simulink library "GOcontroll_Generic"  (R2023b)
settings: Solver=ode45  StartTime=0.0  StopTime=10.0  RelTol=1e-3  EnableMultiTasking=on
undefined symbols (not defined in the file or in its folder): C_CatOutPos, C_Cb1Pt10, Cb1Pt10_RAW_ERR_HIGH, Cb1Pt10_RAW_ERR_LOW, Cb1Pt10_SIG_ERR_HIGH, Cb1Pt10_SIG_ERR_LOW, Cb1Pt10_SIG_WAR_HIGH, Cb1Pt10_SIG_WAR_LOW, M_CatOutPos, Pres_0_20_bar_500_4500_mv_inv, SensorSignalSimulation, signal_x_RAW_ERR_HIGH, signal_x_RAW_ERR_LOW, signal_x_SIG_ERR_HIGH, signal_x_SIG_ERR_LOW, signal_x_SIG_WAR_HIGH, signal_x_SIG_WAR_LOW, signal_x_SPN, Valve1_ACTIVE_DUTY_CYCLE, Valve1_MAX_CURRENT, Valve1_MIN_CURRENT, Valve1_SPN
libraries: simulink x23, GOcontroll_Moduline_Target x20
(part 2 of 2)

== stateflow chart GOcontroll_Generic/Plausability Checks/H2 PPM Diagnose 2 Levels/Chart4 ==
  state Entry
    en:SetDiagnosticCode = 0;
  state System_Running
  state Error_Triggered
  state Error_Triggered_Confirmed
    en:SetDiagnosticCode = 1;
  state Error_Code_Stored
    en:SetDiagnosticCode = 0;
  (default) -> Entry
  Entry -> System_Running : [after(StartupDelayMs,msec)]
  Error_Triggered -> System_Running [order 2] : [Trigger == 0]
  Error_Code_Stored -> System_Running
  System_Running -> Error_Triggered : [Trigger == 1]
  Error_Triggered -> Error_Triggered_Confirmed [order 1] : [after(TriggerDurationMs,msec)]
  Error_Triggered_Confirmed -> Error_Code_Stored : [after(1,sec)]
  data: Trigger input; StartupDelayMs input single; TriggerDurationMs input single; SetDiagnosticCode output uint8

== stateflow chart GOcontroll_Generic/Plausability Checks/Actuator No//Low Current Detection/Chart ==
  state Entry
    en:SetDiagnosticCode = 0;
  state Valve_Actuating
  state Current_Flowing
  state No_Valve_Current
    en:SetDiagnosticCode = 1;
  state Valve_Actuated
  (default) -> Entry
  Valve_Actuated -> Entry [order 2] : [ValveState==0]
  Current_Flowing -> Entry [order 3] : [ValveState==0]
  Valve_Actuating -> Entry [order 1] : [ValveState==0]
  Entry -> Valve_Actuating : [ValveState==1]
  Valve_Actuating -> Current_Flowing [order 2] : [after(100,msec)]
  Current_Flowing -> No_Valve_Current [order 2] : [after(100,msec)]
  Current_Flowing -> Valve_Actuated [order 1] : [ValveCurrent>=MinimalActuatedValveCurrent]
  Valve_Actuated -> No_Valve_Current [order 1] : [ValveCurrent<MinimalActuatedValveCurrent && ValveState==1]
  data: ValveState input; ValveCurrent input; SetDiagnosticCode output; MinimalActuatedValveCurrent parameter

== stateflow chart GOcontroll_Generic/Diagnostic checks/Actuator diagnostic/Chart1 ==
  state Entry
    en:SetDiagnosticCode = 0;
    en:FlagPersist = uint8(0);
    en:FlagVolatile = uint8(0);
  state Reset_Flag
    state System_Running
      en:FlagVolatile = 0;
    state Error_Triggered
    state Error_Triggered_Confirmed
      en:SetDiagnosticCode = 1;
      en:FlagPersist = 1;
      en:FlagVolatile = 1;
    state Error_Code_Stored
      en:SetDiagnosticCode = 0;
    System_Running -> Error_Triggered : [Trigger == 1]
    Error_Triggered -> System_Running [order 2] : [Trigger == 0]
    Error_Code_Stored -> System_Running : [Trigger == 0]
    Error_Triggered -> Error_Triggered_Confirmed [order 1] : [after(duration,msec)]
    Error_Triggered_Confirmed -> Error_Code_Stored : [after(1,sec)]
  (default) -> Entry
  Entry -> System_Running : [after(delay,msec)]
  Reset_Flag -> Entry : [Reset == 1]
  data: Reset input; FlagPersist output; FlagVolatile output; Trigger input; SetDiagnosticCode output uint8; delay parameter single; duration parameter single

== stateflow chart GOcontroll_Generic/Plausability Checks/Actuator short circuit//over current detection/Chart ==
  state DefaultState
    en:SetFaultCode = 0;
  state AlertState
  state ErrorState
    en:SetFaultCode = 1;
  (default) -> DefaultState
  AlertState -> DefaultState [order 1] : [Trigger==0]
  DefaultState -> AlertState : [Trigger==1]
  AlertState -> ErrorState [order 2] : [after(2,sec)]
  data: Trigger input; SetFaultCode output

== stateflow chart GOcontroll_Generic/Plausability Checks/Actuator short circuit//over current detection/Chart1 ==
  state DefaultState
    en:SetFaultCode = 0;
  state AlertState
  state ErrorState
    en:SetFaultCode = 1;
  (default) -> DefaultState
  AlertState -> DefaultState [order 1] : [Trigger==0]
  DefaultState -> AlertState : [Trigger==1]
  AlertState -> ErrorState [order 2] : [after(2,sec)]
  data: Trigger input; SetFaultCode output

== stateflow chart GOcontroll_Generic/Diagnostic checks/Actuator diagnostic/Chart4 ==
  state Entry
    en:SetDiagnosticCode = 0;
    en:FlagPersist = uint8(0);
    en:FlagVolatile = uint8(0);
  state Reset_Flag
    state System_Running
      en:FlagVolatile = 0;
    state Error_Triggered
    state Error_Triggered_Confirmed
      en:SetDiagnosticCode = 1;
      en:FlagPersist = 1;
      en:FlagVolatile = 1;
    state Error_Code_Stored
      en:SetDiagnosticCode = 0;
    System_Running -> Error_Triggered : [Trigger == 1]
    Error_Triggered -> System_Running [order 2] : [Trigger == 0]
    Error_Code_Stored -> System_Running : [Trigger == 0]
    Error_Triggered -> Error_Triggered_Confirmed [order 1] : [after(duration,msec)]
    Error_Triggered_Confirmed -> Error_Code_Stored : [after(1,sec)]
  (default) -> Entry
  Entry -> System_Running : [after(delay,msec)]
  Reset_Flag -> Entry : [Reset == 1]
  data: Reset input; FlagPersist output; FlagVolatile output; Trigger input; SetDiagnosticCode output uint8; delay parameter single; duration parameter single

== stateflow chart GOcontroll_Generic/Diagnostic checks/Generic diagnostic/Chart4 ==
  state Entry
    en:SetDiagnosticCode = 0;
    en:FlagPersist = uint8(0);
    en:FlagVolatile = uint8(0);
  state Reset_Flag
    state System_Running
      en:FlagVolatile = 0;
    state Error_Triggered
    state Error_Triggered_Confirmed
      en:SetDiagnosticCode = 1;
      en:FlagPersist = 1;
      en:FlagVolatile = 1;
    state Error_Code_Stored
      en:SetDiagnosticCode = 0;
    System_Running -> Error_Triggered : [Trigger == 1]
    Error_Triggered -> System_Running [order 2] : [Trigger == 0]
    Error_Code_Stored -> System_Running : [Trigger == 0]
    Error_Triggered -> Error_Triggered_Confirmed [order 1] : [after(duration,msec)]
    Error_Triggered_Confirmed -> Error_Code_Stored : [after(1,sec)]
  (default) -> Entry
  Entry -> System_Running : [after(delay,msec)]
  Reset_Flag -> Entry : [Reset == 1]
  data: Reset input; FlagPersist output; FlagVolatile output; Trigger input; SetDiagnosticCode output uint8; delay parameter single; duration parameter single

== stateflow chart GOcontroll_Generic/Plausability Checks/Tank Pressure & Temp Diagnostic Block/Chart10 ==
  state Entry
    en:SetDiagnosticCode = 0;
  state System_Running
  state Error_Triggered
  state Error_Triggered_Confirmed
    en:SetDiagnosticCode = 1;
  state Error_Code_Stored
    en:SetDiagnosticCode = 0;
  (default) -> Entry
  Entry -> System_Running : [after(StartupDelayMs,msec)]
  Error_Triggered -> System_Running [order 2] : [Trigger == 0]
  Error_Code_Stored -> System_Running
  System_Running -> Error_Triggered : [Trigger == 1]
  Error_Triggered -> Error_Triggered_Confirmed [order 1] : [after(TriggerDurationMs,msec)]
  Error_Triggered_Confirmed -> Error_Code_Stored : [after(1,sec)]
  data: Trigger input; StartupDelayMs input single; TriggerDurationMs input single; SetDiagnosticCode output uint8

== stateflow chart GOcontroll_Generic/Diagnostic checks/Signal diagnostic/Chart1 ==
  state Entry
    en:SetDiagnosticCode = 0;
    en:FlagPersist = 0;
    en:FlagVolatile = 0;
  state Reset_Flag
    state System_Running
      en:FlagVolatile = 0;
    state Error_Triggered
    state Error_Triggered_Confirmed
      en:SetDiagnosticCode = 1;
      en:FlagPersist = 1;
      en:FlagVolatile = 1;
    state Error_Code_Stored
      en:SetDiagnosticCode = 0;
    System_Running -> Error_Triggered : [Trigger == 1]
    Error_Triggered -> System_Running [order 2] : [Trigger == 0]
    Error_Code_Stored -> System_Running : [Trigger == 0]
    Error_Triggered -> Error_Triggered_Confirmed [order 1] : [after(duration,msec)]
    Error_Triggered_Confirmed -> Error_Code_Stored : [after(1,sec)]
  (default) -> Entry
  Entry -> System_Running : [after(delay,msec)]
  Reset_Flag -> Entry : [Reset == 1]
  data: Reset input; FlagPersist output; FlagVolatile output; Trigger input; SetDiagnosticCode output uint8; delay parameter single; duration parameter single

== stateflow chart GOcontroll_Generic/Plausability Checks/Chart4 ==
  state Entry
    en:SetDiagnosticCode = 0;
  state System_Running
  state Error_Triggered
  state Error_Triggered_Confirmed
    en:SetDiagnosticCode = 1;
  state Error_Code_Stored
    en:SetDiagnosticCode = 0;
  (default) -> Entry
  Entry -> System_Running : [after(StartupDelayMs,msec)]
  Error_Triggered -> System_Running [order 2] : [Trigger == 0]
  Error_Code_Stored -> System_Running
  System_Running -> Error_Triggered : [Trigger == 1]
  Error_Triggered -> Error_Triggered_Confirmed [order 1] : [after(TriggerDurationMs,msec)]
  Error_Triggered_Confirmed -> Error_Code_Stored : [after(1,sec)]
  data: Trigger input; StartupDelayMs input single; TriggerDurationMs input single; SetDiagnosticCode output uint8

== stateflow chart GOcontroll_Generic/Diagnostic checks/Signal diagnostic/Chart2 ==
  state Entry
    en:SetDiagnosticCode = 0;
    en:FlagPersist = 0;
    en:FlagVolatile = 0;
  state Reset_Flag
    state System_Running
      en:FlagVolatile = 0;
    state Error_Triggered
    state Error_Triggered_Confirmed
      en:SetDiagnosticCode = 1;
      en:FlagPersist = 1;
      en:FlagVolatile = 1;
    state Error_Code_Stored
      en:SetDiagnosticCode = 0;
    System_Running -> Error_Triggered : [Trigger == 1]
    Error_Triggered -> System_Running [order 2] : [Trigger == 0]
    Error_Code_Stored -> System_Running : [Trigger == 0]
    Error_Triggered -> Error_Triggered_Confirmed [order 1] : [after(duration,msec)]
    Error_Triggered_Confirmed -> Error_Code_Stored : [after(1,sec)]
  (default) -> Entry
  Entry -> System_Running : [after(delay,msec)]
  Reset_Flag -> Entry : [Reset == 1]
  data: Reset input; FlagPersist output; FlagVolatile output; Trigger input; SetDiagnosticCode output uint8; delay parameter single; duration parameter single

== stateflow chart GOcontroll_Generic/Diagnostic checks/Signal diagnostic/Chart3 ==
  state Entry
    en:SetDiagnosticCode = 0;
    en:FlagPersist = 0;
    en:FlagVolatile = 0;
  state Reset_Flag
    state System_Running
      en:FlagVolatile = 0;
    state Error_Triggered
    state Error_Triggered_Confirmed
      en:SetDiagnosticCode = 1;
      en:FlagPersist = 1;
      en:FlagVolatile = 1;
    state Error_Code_Stored
      en:SetDiagnosticCode = 0;
    System_Running -> Error_Triggered : [Trigger == 1]
    Error_Triggered -> System_Running [order 2] : [Trigger == 0]
    Error_Code_Stored -> System_Running : [Trigger == 0]
    Error_Triggered -> Error_Triggered_Confirmed [order 1] : [after(duration,msec)]
    Error_Triggered_Confirmed -> Error_Code_Stored : [after(1,sec)]
  (default) -> Entry
  Entry -> System_Running : [after(delay,msec)]
  Reset_Flag -> Entry : [Reset == 1]
  data: Reset input; FlagPersist output; FlagVolatile output; Trigger input; SetDiagnosticCode output uint8; delay parameter single; duration parameter single

== stateflow chart GOcontroll_Generic/Diagnostic checks/Signal diagnostic/Chart4 ==
  state Entry
    en:SetDiagnosticCode = 0;
    en:FlagPersist = 0;
    en:FlagVolatile = 0;
  state Reset_Flag
    state System_Running
      en:FlagVolatile = 0;
    state Error_Triggered
    state Error_Triggered_Confirmed
      en:SetDiagnosticCode = 1;
      en:FlagPersist = 1;
      en:FlagVolatile = 1;
    state Error_Code_Stored
      en:SetDiagnosticCode = 0;
    System_Running -> Error_Triggered : [Trigger == 1]
    Error_Triggered -> System_Running [order 2] : [Trigger == 0]
    Error_Code_Stored -> System_Running : [Trigger == 0]
    Error_Triggered -> Error_Triggered_Confirmed [order 1] : [after(duration,msec)]
    Error_Triggered_Confirmed -> Error_Code_Stored : [after(1,sec)]
  (default) -> Entry
  Entry -> System_Running : [after(delay,msec)]
  Reset_Flag -> Entry : [Reset == 1]
  data: Reset input; FlagPersist output; FlagVolatile output; Trigger input; SetDiagnosticCode output uint8; delay parameter single; duration parameter single

== stateflow chart GOcontroll_Generic/Diagnostic checks/Signal diagnostic/Chart5 ==
  state Entry
    en:SetDiagnosticCode = 0;
    en:FlagPersist = 0;
    en:FlagVolatile = 0;
  state Reset_Flag
    state System_Running
      en:FlagVolatile = 0;
    state Error_Triggered
    state Error_Triggered_Confirmed
      en:SetDiagnosticCode = 1;
      en:FlagPersist = 1;
      en:FlagVolatile = 1;
    state Error_Code_Stored
      en:SetDiagnosticCode = 0;
    System_Running -> Error_Triggered : [Trigger == 1]
    Error_Triggered -> System_Running [order 2] : [Trigger == 0]
    Error_Code_Stored -> System_Running : [Trigger == 0]
    Error_Triggered -> Error_Triggered_Confirmed [order 1] : [after(duration,msec)]
    Error_Triggered_Confirmed -> Error_Code_Stored : [after(1,sec)]
  (default) -> Entry
  Entry -> System_Running : [after(delay,msec)]
  Reset_Flag -> Entry : [Reset == 1]
  data: Reset input; FlagPersist output; FlagVolatile output; Trigger input; SetDiagnosticCode output uint8; delay parameter single; duration parameter single

== stateflow chart GOcontroll_Generic/Diagnostic checks/Signal diagnostic/Chart6 ==
  state Entry
    en:SetDiagnosticCode = 0;
    en:FlagPersist = 0;
    en:FlagVolatile = 0;
  state Reset_Flag
    state System_Running
      en:FlagVolatile = 0;
    state Error_Triggered
    state Error_Triggered_Confirmed
      en:SetDiagnosticCode = 1;
      en:FlagPersist = 1;
      en:FlagVolatile = 1;
    state Error_Code_Stored
      en:SetDiagnosticCode = 0;
    System_Running -> Error_Triggered : [Trigger == 1]
    Error_Triggered -> System_Running [order 2] : [Trigger == 0]
    Error_Code_Stored -> System_Running : [Trigger == 0]
    Error_Triggered -> Error_Triggered_Confirmed [order 1] : [after(duration,msec)]
    Error_Triggered_Confirmed -> Error_Code_Stored : [after(1,sec)]
  (default) -> Entry
  Entry -> System_Running : [after(delay,msec)]
  Reset_Flag -> Entry : [Reset == 1]
  data: Reset input; FlagPersist output; FlagVolatile output; Trigger input; SetDiagnosticCode output uint8; delay parameter single; duration parameter single

== stateflow chart GOcontroll_Generic/Plausability Checks/Tank Pressure & Temp Diagnostic Block/Chart5 ==
  state Entry
    en:SetDiagnosticCode = 0;
  state System_Running
  state Error_Triggered
  state Error_Triggered_Confirmed
    en:SetDiagnosticCode = 1;
  state Error_Code_Stored
    en:SetDiagnosticCode = 0;
  (default) -> Entry
  Entry -> System_Running : [after(StartupDelayMs,msec)]
  Error_Triggered -> System_Running [order 2] : [Trigger == 0]
  Error_Code_Stored -> System_Running
  System_Running -> Error_Triggered : [Trigger == 1]
  Error_Triggered -> Error_Triggered_Confirmed [order 1] : [after(TriggerDurationMs,msec)]
  Error_Triggered_Confirmed -> Error_Code_Stored : [after(1,sec)]
  data: Trigger input; StartupDelayMs input single; TriggerDurationMs input single; SetDiagnosticCode output uint8

== stateflow chart GOcontroll_Generic/Plausability Checks/Tank Pressure & Temp Diagnostic Block/Chart6 ==
  state Entry
    en:SetDiagnosticCode = 0;
  state System_Running
  state Error_Triggered
  state Error_Triggered_Confirmed
    en:SetDiagnosticCode = 1;
  state Error_Code_Stored
    en:SetDiagnosticCode = 0;
  (default) -> Entry
  Entry -> System_Running : [after(StartupDelayMs,msec)]
  Error_Triggered -> System_Running [order 2] : [Trigger == 0]
  Error_Code_Stored -> System_Running
  System_Running -> Error_Triggered : [Trigger == 1]
  Error_Triggered -> Error_Triggered_Confirmed [order 1] : [after(TriggerDurationMs,msec)]
  Error_Triggered_Confirmed -> Error_Code_Stored : [after(1,sec)]
  data: Trigger input; StartupDelayMs input single; TriggerDurationMs input single; SetDiagnosticCode output uint8

== stateflow chart GOcontroll_Generic/Plausability Checks/Tank Pressure & Temp Diagnostic Block/Chart7 ==
  state Entry
    en:SetDiagnosticCode = 0;
  state System_Running
  state Error_Triggered
  state Error_Triggered_Confirmed
    en:SetDiagnosticCode = 1;
  state Error_Code_Stored
    en:SetDiagnosticCode = 0;
  (default) -> Entry
  Entry -> System_Running : [after(StartupDelayMs,msec)]
  Error_Triggered -> System_Running [order 2] : [Trigger == 0]
  Error_Code_Stored -> System_Running
  System_Running -> Error_Triggered : [Trigger == 1]
  Error_Triggered -> Error_Triggered_Confirmed [order 1] : [after(TriggerDurationMs,msec)]
  Error_Triggered_Confirmed -> Error_Code_Stored : [after(1,sec)]
  data: Trigger input; StartupDelayMs input single; TriggerDurationMs input single; SetDiagnosticCode output uint8
